simulink model "Test3C120Board_HSMA"  (Simulink 7.1)
settings: Solver=ode45  SolverMode=SingleTasking  StartTime=0.0  StopTime=1000.0  FixedStep=1  RelTol=1e-3
InitFcn:
  | %% DSPBuilder Start
  | alt_dspbuilder_update_model(bdroot)
  | %% DSPBuilder End
undefined symbols (not defined in the file): Pin_AB1, Pin_AB2, Pin_AB6, Pin_AC5, Pin_AE3, Pin_AF2, Pin_F4, Pin_F5, Pin_G1, Pin_G2, Pin_G3, Pin_G4, Pin_H3, Pin_H4, Pin_J3, Pin_J4, Pin_J5, Pin_J6, Pin_J7, Pin_K1, Pin_K2, Pin_K3, Pin_K4, Pin_K7, Pin_K8, Pin_L1, Pin_L2, Pin_L3, Pin_L4, Pin_L6, Pin_L7, Pin_L8, Pin_M7, Pin_M8, Pin_N3, Pin_N4, Pin_P1, Pin_P2, Pin_R3, Pin_R4, Pin_R6, Pin_R7, Pin_T3, Pin_T4, Pin_U1, Pin_U2, Pin_U3, Pin_U4, Pin_V1, Pin_V2, Pin_V3, Pin_V4, Pin_W1, Pin_W2, Pin_Y3, Pin_Y4
libraries: allblocks_alteradspbuilder2 x50, Cyclone_III_EP3C120_alteradspbuilder2 x5
settings Model: Creator=lkong  LastModifiedBy=lkong
settings DataIOCC: SignalLoggingName=sigsOut
settings OptimizationCC: InlineInvariantSignals=on
settings DebuggingCC: SaveWithParameterizedLinksMsg=none  SignalResolutionControl=TryResolveAllWithWarning  SolverPrmCheckMsg=none  MultiTaskDSMMsg=warning  MultiTaskCondExecSysMsg=none  StrictBusMsg=None
settings HardwareCC: TargetUnknown=on
settings RTWCC: IncludeERTFirstTime=on
settings GRTTargetCC: TargetFcnLib=ansi_tfl_tmw.mat  ModelReferenceCompliant=off  MatFileLogging=off

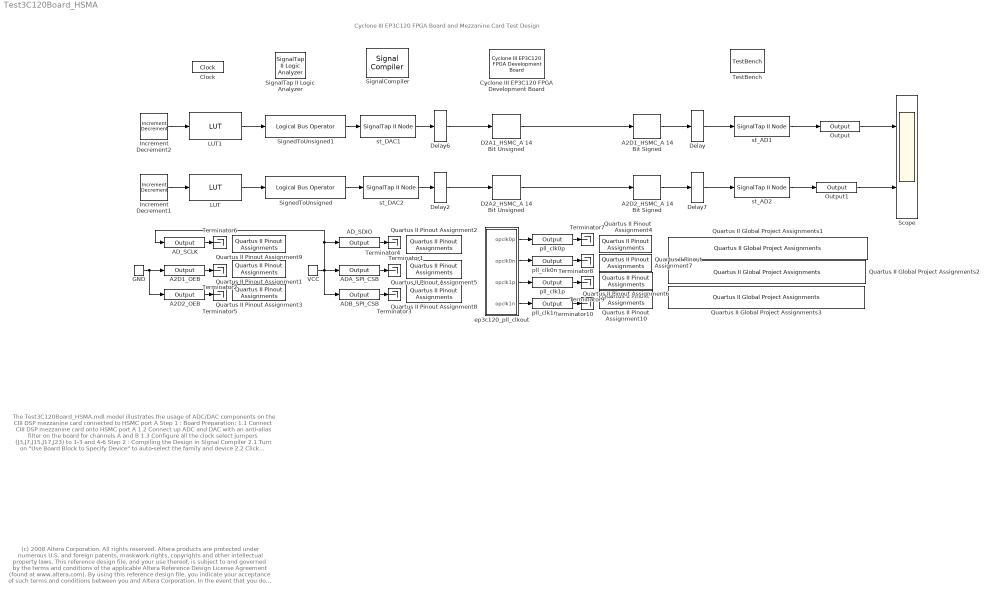
== system Test3C120Board_HSMA ==
  note: Cyclone III EP3C120 FPGA Board and Mezzanine Card Test Design
  note: (c) 2008 Altera Corporation. All rights reserved.  Altera products are protected under numerous U.S. and foreign patents, maskwork rights, copyrights and other intellectual property laws.
      | This reference design file, and your use thereof, is subject to and governed by the terms and conditions of the applicable Altera Reference Design License Agreement (found at www.altera.com).
      | By using this reference design file, you indicate your acceptance of such terms and conditions between you and Altera Corporation.
      | In the event that you do not agree with such terms and conditions, you may not use the reference design file and please promptly destroy any copies you have made.
      | This reference design file being provided on an "as-is" basis and as an accommodation and therefore all warranties, representations or guarantees of any kind (whether express, implied or statutory)
      | including, without limitation, warranties of merchantability, non-infringement, or fitness for a particular purpose, are specifically disclaimed.
      | By making this reference design file available, Altera expressly does not recommend, suggest or require that this reference design file be used in combination with any other product not provided by Altera
  note: The Test3C120Board_HSMA.mdl model illustrates the usage of ADC/DAC components on the CIII DSP mezzanine card connected to HSMC port A
      |
      | Step 1 : Board Preparation:
      |                1.1 Connect CIII DSP mezzanine card onto HSMC port A
      |                1.2 Connect up ADC and DAC with an anti-alias filter on the board for channels A and B
      |                1.3 Configure all the clock select jumpers (J3,J7,J15,J17,J23) to 1-3 and 4-6
      | Step 2 : Compiling the Design in Signal Compiler
      |                2.1 Turn on "Use Board Block to Specify Device" to auto-select the family and device
      |                2.2 Click "Compile" to compile the design through the Quartus II software and create a .sof file
      |                2.3 Click "Scan Jtag" to select a download cable and device
      |                2.4 Click "Program" to download the .sof file onto the FPGA device
      | Step 3 : Running SignalTap II Logic Analyzer
      |                3.1 Click "Scan Jtag" to select a download cable and device
      |                3.2 Click "Acquire" to obtain data for embedded SignalTap II nodes
  A2D1_HSMC_A 14 Bit Signed : Cyclone_III_EP3C120_alteradspbuilder2/A2D1_HSMC_A 14 Bit Signed  iofile=D:\dspbuilder\dspb91\ShippedDesignExamples\tb_Test3C120Board_HSMA\Test3C120Board%5FHSMA_A2D1%5FHSMC%5FA+14+Bit+Signed.salt  externalType=Inferred  SpecifyClock=off  location=Pin_P1,Pin_P2,Pin_M7,Pin_M8,Pin_R4,Pin_R3,Pin_T3,Pin_T4,Pin_V3,Pin_V4,Pin_R6,Pin_R7,Pin_AE3,Pin_AB6
  A2D1_OEB : allblocks_alteradspbuilder2/Output  iofile=D:\dspbuilder\dspb91\ShippedDesignExamples\tb_Test3C120Board_HSMA\Test3C120Board%5FHSMA_A2D1%5FOEB.capture  BusType=Single Bit  bwl=1  bwr=0  externalType=Inferred  PORTTYPE=Output  allowFloatingPointOverride=on  logOutputs=off
  A2D2_HSMC_A 14 Bit Signed : Cyclone_III_EP3C120_alteradspbuilder2/A2D2_HSMC_A 14 Bit Signed  iofile=D:\dspbuilder\dspb91\ShippedDesignExamples\tb_Test3C120Board_HSMA\Test3C120Board%5FHSMA_A2D2%5FHSMC%5FA+14+Bit+Signed.salt  externalType=Inferred  SpecifyClock=off  location=Pin_U1,Pin_U2,Pin_V1,Pin_V2,Pin_W1,Pin_W2,Pin_U4,Pin_U3,Pin_Y3,Pin_Y4,Pin_AB1,Pin_AB2,Pin_AC5,Pin_AF2
  A2D2_OEB : allblocks_alteradspbuilder2/Output  iofile=D:\dspbuilder\dspb91\ShippedDesignExamples\tb_Test3C120Board_HSMA\Test3C120Board%5FHSMA_A2D2%5FOEB.capture  BusType=Single Bit  bwl=1  bwr=0  externalType=Inferred  PORTTYPE=Output  allowFloatingPointOverride=on  logOutputs=off
  ADA_SPI_CSB : allblocks_alteradspbuilder2/Output  iofile=D:\dspbuilder\dspb91\ShippedDesignExamples\tb_Test3C120Board_HSMA\Test3C120Board%5FHSMA_ADA%5FSPI%5FCSB.capture  BusType=Single Bit  bwl=1  bwr=0  externalType=Inferred  PORTTYPE=Output  allowFloatingPointOverride=on  logOutputs=off
  ADB_SPI_CSB : allblocks_alteradspbuilder2/Output  iofile=D:\dspbuilder\dspb91\ShippedDesignExamples\tb_Test3C120Board_HSMA\Test3C120Board%5FHSMA_ADB%5FSPI%5FCSB.capture  BusType=Single Bit  bwl=1  bwr=0  externalType=Inferred  PORTTYPE=Output  allowFloatingPointOverride=on  logOutputs=off
  AD_SCLK : allblocks_alteradspbuilder2/Output  iofile=D:\dspbuilder\dspb91\ShippedDesignExamples\tb_Test3C120Board_HSMA\Test3C120Board%5FHSMA_AD%5FSCLK.capture  BusType=Single Bit  bwl=1  bwr=0  externalType=Inferred  PORTTYPE=Output  allowFloatingPointOverride=on  logOutputs=off
  AD_SDIO : allblocks_alteradspbuilder2/Output  iofile=D:\dspbuilder\dspb91\ShippedDesignExamples\tb_Test3C120Board_HSMA\Test3C120Board%5FHSMA_AD%5FSDIO.capture  BusType=Single Bit  bwl=1  bwr=0  externalType=Inferred  PORTTYPE=Output  allowFloatingPointOverride=on  logOutputs=off
  Clock : allblocks_alteradspbuilder2/Clock  ClockPeriod=20  ClockPeriodUnit=ns  SampleTime=1  ResetLatency=0  ResetRegisterCascadeDepth=0  SimulationStartCycle=5  PhaseOffset=0  Reset=aclr  ResetType=Active Low  Export=off
  Cyclone III EP3C120 FPGA Development Board : Cyclone_III_EP3C120_alteradspbuilder2/Cyclone III EP3C120 FPGA Development Board  ClockPinIn=Pin_AH15  GlobalResetPin=Pin_T21  device=EP3C120F780C7
  D2A1_HSMC_A 14 Bit Unsigned : Cyclone_III_EP3C120_alteradspbuilder2/D2A1_HSMC_A 14 Bit Unsigned  iofile=D:\dspbuilder\dspb91\ShippedDesignExamples\tb_Test3C120Board_HSMA\Test3C120Board%5FHSMA_D2A1%5FHSMC%5FA+14+Bit+Unsigned.capture  externalType=Inferred  location=Pin_F4,Pin_F5,Pin_G1,Pin_G2,Pin_K7,Pin_J7,Pin_J3,Pin_J4,Pin_K3,Pin_K4,Pin_L8,Pin_K8,Pin_L6,Pin_L7
  D2A2_HSMC_A 14 Bit Unsigned : Cyclone_III_EP3C120_alteradspbuilder2/D2A2_HSMC_A 14 Bit Unsigned  iofile=D:\dspbuilder\dspb91\ShippedDesignExamples\tb_Test3C120Board_HSMA\Test3C120Board%5FHSMA_D2A2%5FHSMC%5FA+14+Bit+Unsigned.capture  externalType=Inferred  location=Pin_G3,Pin_G4,Pin_H3,Pin_H4,Pin_J5,Pin_J6,Pin_K1,Pin_K2,Pin_L1,Pin_L2,Pin_L3,Pin_L4,Pin_N3,Pin_N4
  Delay : allblocks_alteradspbuilder2/Delay  pipeline=1  pipeline_display=1  ClockPhase=1  use_ena=off  use_sclr=off  allowFloatingPointOverride=on  logOutputs=off  logFile=D:\dspbuilder\dspb91\ShippedDesignExamples\tb_Test3C120Board_HSMA\Test3C120Board%5FHSMA_Delay.fixedpointlog  use_init=off  reset_value=1
  Delay2 : allblocks_alteradspbuilder2/Delay  pipeline=1  pipeline_display=1  ClockPhase=1  use_ena=off  use_sclr=off  allowFloatingPointOverride=on  logOutputs=off  logFile=D:\dspbuilder\dspb91\ShippedDesignExamples\tb_Test3C120Board_HSMA\Test3C120Board%5FHSMA_Delay2.fixedpointlog  use_init=off  reset_value=1
  Delay6 : allblocks_alteradspbuilder2/Delay  pipeline=1  pipeline_display=1  ClockPhase=1  use_ena=off  use_sclr=off  allowFloatingPointOverride=on  logOutputs=off  logFile=D:\dspbuilder\dspb91\ShippedDesignExamples\tb_Test3C120Board_HSMA\Test3C120Board%5FHSMA_Delay6.fixedpointlog  use_init=off  reset_value=1
  Delay7 : allblocks_alteradspbuilder2/Delay  pipeline=1  pipeline_display=1  ClockPhase=1  use_ena=off  use_sclr=off  allowFloatingPointOverride=on  logOutputs=off  logFile=D:\dspbuilder\dspb91\ShippedDesignExamples\tb_Test3C120Board_HSMA\Test3C120Board%5FHSMA_Delay7.fixedpointlog  use_init=off  reset_value=1
  GND : allblocks_alteradspbuilder2/GND  SpecifyClock=off
  Increment Decrement1 : allblocks_alteradspbuilder2/Increment Decrement  BusType=Unsigned Integer  bwl=7  bwr=0  SpecifyClock=off  clr_value=0  direction=Increment  phase_selection=1  use_ena=off  use_sclr=off  pipeline_display=1
  Increment Decrement2 : allblocks_alteradspbuilder2/Increment Decrement  BusType=Unsigned Integer  bwl=7  bwr=0  SpecifyClock=off  clr_value=0  direction=Increment  phase_selection=1  use_ena=off  use_sclr=off  pipeline_display=1
  LUT : allblocks_alteradspbuilder2/LUT  addr_width=7  BusType=Signed Integer  bwl=14  bwr=0  init_array=8191*sin( [0:2*pi/(2^7):2*pi] )  allowFloatingPointOverride=on  logOutputs=off  logFile=D:\dspbuilder\dspb91\ShippedDesignExamples\tb_Test3C120Board_HSMA\Test3C120Board%5FHSMA_LUT.fixedpointlog  use_ena=off  reg_data=on  use_lpm=on  reg_addr=on  ram_type=AUTO  pipeline_display=2
  LUT1 : allblocks_alteradspbuilder2/LUT  addr_width=7  BusType=Signed Integer  bwl=14  bwr=0  init_array=8191*sin( [0:2*pi/(2^7):2*pi] )  allowFloatingPointOverride=on  logOutputs=off  logFile=D:\dspbuilder\dspb91\ShippedDesignExamples\tb_Test3C120Board_HSMA\Test3C120Board%5FHSMA_LUT1.fixedpointlog  use_ena=off  reg_data=on  use_lpm=on  reg_addr=on  ram_type=AUTO  pipeline_display=2
  Output : allblocks_alteradspbuilder2/Output  iofile=D:\dspbuilder\dspb91\ShippedDesignExamples\tb_Test3C120Board_HSMA\Test3C120Board%5FHSMA_Output.capture  BusType=Unsigned Integer  bwl=14  bwr=0  externalType=Inferred  PORTTYPE=Output  allowFloatingPointOverride=on  logOutputs=off
  Output1 : allblocks_alteradspbuilder2/Output  iofile=D:\dspbuilder\dspb91\ShippedDesignExamples\tb_Test3C120Board_HSMA\Test3C120Board%5FHSMA_Output1.capture  BusType=Signed Integer  bwl=14  bwr=0  externalType=Inferred  PORTTYPE=Output  allowFloatingPointOverride=on  logOutputs=off
  Quartus II Global Project Assignments1 : allblocks_alteradspbuilder2/Quartus II Global Project Assignments  QuartusIIAssignmentName=RESERVE_DATA1_AFTER_CONFIGURATION  QuartusIIAssignmentValue="\"USE AS REGULAR IO\""
  Quartus II Global Project Assignments2 : allblocks_alteradspbuilder2/Quartus II Global Project Assignments  QuartusIIAssignmentName=CYCLONEII_RESERVE_NCEO_AFTER_CONFIGURATION  QuartusIIAssignmentValue="\"USE AS REGULAR IO\""
  Quartus II Global Project Assignments3 : allblocks_alteradspbuilder2/Quartus II Global Project Assignments  QuartusIIAssignmentName=RESERVE_DCLK_AFTER_CONFIGURATION  QuartusIIAssignmentValue="\"USE AS REGULAR IO\""
  Quartus II Pinout Assignment1 : allblocks_alteradspbuilder2/Quartus II Pinout Assignments  QuartusIIAssignmentName=A2D1_OEB  QuartusIIAssignmentValue=Pin_M3
  Quartus II Pinout Assignment10 : allblocks_alteradspbuilder2/Quartus II Pinout Assignments  QuartusIIAssignmentName=pll_clk1n  QuartusIIAssignmentValue=Pin_D1
  Quartus II Pinout Assignment2 : allblocks_alteradspbuilder2/Quartus II Pinout Assignments  QuartusIIAssignmentName=AD_SDIO  QuartusIIAssignmentValue=Pin_M1
  Quartus II Pinout Assignment3 : allblocks_alteradspbuilder2/Quartus II Pinout Assignments  QuartusIIAssignmentName=A2D2_OEB  QuartusIIAssignmentValue=Pin_U5
  Quartus II Pinout Assignment4 : allblocks_alteradspbuilder2/Quartus II Pinout Assignments  QuartusIIAssignmentName=pll_clk0p  QuartusIIAssignmentValue=Pin_G6
  Quartus II Pinout Assignment5 : allblocks_alteradspbuilder2/Quartus II Pinout Assignments  QuartusIIAssignmentName=ADA_SPI_CSB  QuartusIIAssignmentValue=Pin_M2
  Quartus II Pinout Assignment6 : allblocks_alteradspbuilder2/Quartus II Pinout Assignments  QuartusIIAssignmentName=pll_clk1p  QuartusIIAssignmentValue=Pin_D2
  Quartus II Pinout Assignment7 : allblocks_alteradspbuilder2/Quartus II Pinout Assignments  QuartusIIAssignmentName=pll_clk0n  QuartusIIAssignmentValue=Pin_G5
  Quartus II Pinout Assignment8 : allblocks_alteradspbuilder2/Quartus II Pinout Assignments  QuartusIIAssignmentName=ADB_SPI_CSB  QuartusIIAssignmentValue=Pin_R2
  Quartus II Pinout Assignment9 : allblocks_alteradspbuilder2/Quartus II Pinout Assignments  QuartusIIAssignmentName=AD_SCLK  QuartusIIAssignmentValue=Pin_R1
  Scope : Scope  NumInputPorts=2
      settings: YMin=-5~-5  YMax=5~5  SampleInput=on
  SignalCompiler : allblocks_alteradspbuilder2/Signal Compiler  DeviceFamily=Cyclone III  DeviceName=EP3C120F780C7  EnableSignalTap=on  SignalTapDepth=512  UseBoardBlock=on  StpUseDefaultClock=on  StpClock=Clock  ExportDir=C:\Documents and Settings\lkong\My Documents
  SignalTap II Logic Analyzer : allblocks_alteradspbuilder2/SignalTap II Logic Analyzer
  SignedToUnsigned : allblocks_alteradspbuilder2/Logical Bus Operator  BusType=Unsigned Integer  bwl=14  bwr=0  LogicalOp_text=XOR  mask_value_num=8192  shift_amount=3  force_sign_ext=off  pipeline_display=0
  SignedToUnsigned1 : allblocks_alteradspbuilder2/Logical Bus Operator  BusType=Unsigned Integer  bwl=14  bwr=0  LogicalOp_text=XOR  mask_value_num=8192  shift_amount=3  force_sign_ext=off  pipeline_display=0
  Terminator{1..10} (10 alike) : Terminator
  TestBench : allblocks_alteradspbuilder2/TestBench  enable=on  advancedMode=off  modelSimGui=on  maxDisplayErrors=10  mismatchErrorLevel=Error  simdatafile=D:\dspbuilder\dspb91\ShippedDesignExamples\tb_Test3C120Board_HSMA\Test3C120Board_HSMA.simdata.tcl
  VCC : allblocks_alteradspbuilder2/VCC  SpecifyClock=off
  ep3c120_pll_clkout : Subsystem
      mask Type: SubSystem AlteraBlockSet
  pll_clk0n : allblocks_alteradspbuilder2/Output  iofile=D:\dspbuilder\dspb91\ShippedDesignExamples\tb_Test3C120Board_HSMA\Test3C120Board%5FHSMA_pll%5Fclk0n.capture  BusType=Single Bit  bwl=1  bwr=0  externalType=Inferred  PORTTYPE=Output  allowFloatingPointOverride=on  logOutputs=off
  pll_clk0p : allblocks_alteradspbuilder2/Output  iofile=D:\dspbuilder\dspb91\ShippedDesignExamples\tb_Test3C120Board_HSMA\Test3C120Board%5FHSMA_pll%5Fclk0p.capture  BusType=Single Bit  bwl=1  bwr=0  externalType=Inferred  PORTTYPE=Output  allowFloatingPointOverride=on  logOutputs=off
  pll_clk1n : allblocks_alteradspbuilder2/Output  iofile=D:\dspbuilder\dspb91\ShippedDesignExamples\tb_Test3C120Board_HSMA\Test3C120Board%5FHSMA_pll%5Fclk1n.capture  BusType=Single Bit  bwl=1  bwr=0  externalType=Inferred  PORTTYPE=Output  allowFloatingPointOverride=on  logOutputs=off
  pll_clk1p : allblocks_alteradspbuilder2/Output  iofile=D:\dspbuilder\dspb91\ShippedDesignExamples\tb_Test3C120Board_HSMA\Test3C120Board%5FHSMA_pll%5Fclk1p.capture  BusType=Single Bit  bwl=1  bwr=0  externalType=Inferred  PORTTYPE=Output  allowFloatingPointOverride=on  logOutputs=off
  st_AD1 : allblocks_alteradspbuilder2/SignalTap II Node  id=0
  st_AD2 : allblocks_alteradspbuilder2/SignalTap II Node  id=1
  st_DAC1 : allblocks_alteradspbuilder2/SignalTap II Node  id=2
  st_DAC2 : allblocks_alteradspbuilder2/SignalTap II Node  id=3
  wires:
  SignedToUnsigned1/1 -> st_DAC1/1
  Delay/1 -> st_AD1/1
  Delay6/1 -> D2A1_HSMC_A 14 Bit Unsigned/1
  st_DAC1/1 -> Delay6/1
  D2A1_HSMC_A 14 Bit Unsigned/1 -> A2D1_HSMC_A 14 Bit Signed/1
  LUT/1 -> SignedToUnsigned/1
  SignedToUnsigned/1 -> st_DAC2/1
  Increment Decrement1/1 -> LUT/1
  Delay2/1 -> D2A2_HSMC_A 14 Bit Unsigned/1
  st_DAC2/1 -> Delay2/1
  D2A2_HSMC_A 14 Bit Unsigned/1 -> A2D2_HSMC_A 14 Bit Signed/1
  A2D1_HSMC_A 14 Bit Signed/1 -> Delay/1
  A2D2_HSMC_A 14 Bit Signed/1 -> Delay7/1
  Delay7/1 -> st_AD2/1
  st_AD1/1 -> Output/1
  st_AD2/1 -> Output1/1
  Output/1 -> Scope/1
  Output1/1 -> Scope/2
  LUT1/1 -> SignedToUnsigned1/1
  Increment Decrement2/1 -> LUT1/1
  A2D1_OEB/1 -> Terminator2/1
  A2D2_OEB/1 -> Terminator5/1
  GND/1 -> A2D2_OEB/1, A2D1_OEB/1
  ADA_SPI_CSB/1 -> Terminator1/1
  ADB_SPI_CSB/1 -> Terminator3/1
  VCC/1 -> ADB_SPI_CSB/1, ADA_SPI_CSB/1, AD_SDIO/1, AD_SCLK/1
  AD_SDIO/1 -> Terminator4/1
  AD_SCLK/1 -> Terminator6/1
  ep3c120_pll_clkout/1(opclk0p) -> pll_clk0p/1
  ep3c120_pll_clkout/2(opclk0n) -> pll_clk0n/1
  ep3c120_pll_clkout/3(opclk1p) -> pll_clk1p/1
  ep3c120_pll_clkout/4(opclk1n) -> pll_clk1n/1
  pll_clk0p/1 -> Terminator7/1
  pll_clk0n/1 -> Terminator8/1
  pll_clk1p/1 -> Terminator9/1
  pll_clk1n/1 -> Terminator10/1

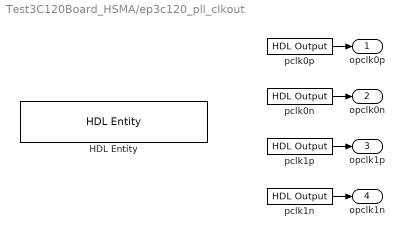
== system Test3C120Board_HSMA/ep3c120_pll_clkout ==
  HDL Entity : allblocks_alteradspbuilder2/HDL Entity  HDLFile=ep3c120_pll_clkout.vhd  clockname=clkin_50  useSubsystemPortName=off
  pclk0n : allblocks_alteradspbuilder2/HDL Output  BusType=Single Bit  bwl=1  bwr=0  externalType=Inferred
  pclk0p : allblocks_alteradspbuilder2/HDL Output  BusType=Single Bit  bwl=1  bwr=0  externalType=Inferred
  pclk1n : allblocks_alteradspbuilder2/HDL Output  BusType=Single Bit  bwl=1  bwr=0  externalType=Inferred
  pclk1p : allblocks_alteradspbuilder2/HDL Output  BusType=Single Bit  bwl=1  bwr=0  externalType=Inferred
  opclk0p : Outport  OutDataType=sfix(16)  OutScaling=2^0
  opclk0n : Outport  Port=2  OutDataType=sfix(16)  OutScaling=2^0
  opclk1p : Outport  Port=3  OutDataType=sfix(16)  OutScaling=2^0
  opclk1n : Outport  Port=4  OutDataType=sfix(16)  OutScaling=2^0
  wires:
  pclk0p/1 -> opclk0p/1
  pclk0n/1 -> opclk0n/1
  pclk1p/1 -> opclk1p/1
  pclk1n/1 -> opclk1n/1
